simulink model "dcmotor_ff"  (R2014b)
settings: Solver=ode45  StartTime=0.0  StopTime=20  FixedStep=1  RelTol=1e-3
PreLoadFcn:
  | param_dcmotor2
values from neighbouring files (symbols this model uses):
  AngleRange = 3500    [param_dcmotor.m]
  Bm = 1e-4    (= 0.0001)    [param_dcmotor.m]
  FN = 620    [param_dcmotor.m]
  J = 0.028 * 1e-4    (= 2.8e-06)    [param_dcmotor.m]
  KD = 8.20 * 1e-5    (= 8.2e-05)    [param_dcmotor.m]
  Ke = 0.0506    [param_dcmotor.m]
  KI = 0.0291    [param_dcmotor.m]
  KP = 0.0136    [param_dcmotor.m]
  Kt = 0.051    [param_dcmotor.m]
  La = 4.4 * 1e-3    (= 0.0044)    [param_dcmotor.m]
  PWMCycle = 10000    [param_dcmotor.m]
  Ra = 10    [param_dcmotor.m]
  TL = 0    [param_dcmotor.m]
  Vol0 = 2.5    [param_dcmotor.m]
  VolMotor = 24    [param_dcmotor.m]
  VolRange = 4.5    [param_dcmotor.m]
undefined symbols (not defined in the file or in its folder): sigbuilder_block
libraries: simulink x2
settings Model: Creator=yyamamot  LastModifiedBy=kotsuka
settings DataIOCC: SignalLoggingSaveFormat=ModelDataLogs  DSMLogging=off
settings OptimizationCC: ExpressionDepthLimit=2147483647  OptimizeModelRefInitCode=on  LifeSpan=1
settings DebuggingCC: UnderspecifiedInitializationDetection=Classic  MergeDetectMultiDrivingBlocksExec=none  ParameterPrecisionLossMsg=none  FcnCallInpInsideContextMsg=UseLocalSettings  StateNameClashWarn=warning
settings HardwareCC: ProdIntDivRoundTo=Zero  ProdEndianess=LittleEndian  ProdHWDeviceType=Generic->32-bit Embedded Processor
settings RTWCC: SystemTargetFile=ert.tlc  GenCodeOnly=on  TemplateMakefile=ert_default_tmf  Description=Real-Time Workshop Embedded Coder  GenerateReport=on  RTWVerbose=off  ProcessScript=ert_make_rtw_hook  IncludeHyperlinkInReport=on  LaunchReport=on  GenerateTraceInfo=on  GenerateTraceReport=on  GenerateTraceReportSl=on  GenerateTraceReportSf=on  GenerateTraceReportEml=on
settings CodeAppCC: IgnoreCustomStorageClasses=off  CustomSymbolStrType=$N$R$M  InternalIdentifier=Classic
settings ERTTargetCC: GenerateSampleERTMain=on  IncludeMdlTerminateFcn=off  SuppressErrorStatus=on  SupportAbsoluteTime=off  SupportNonFinite=off  SupportComplex=off  ERTCustomFileTemplate=example_file_process.tlc

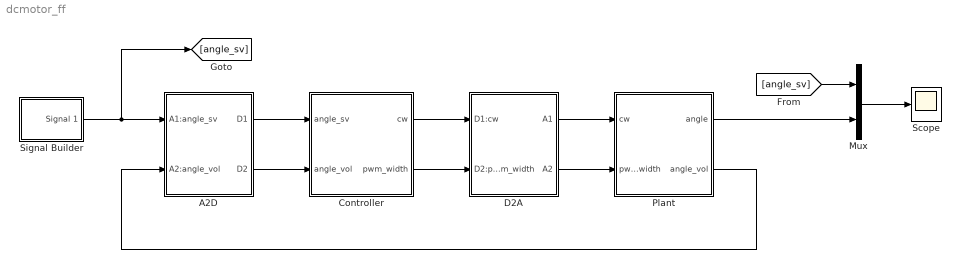
== system dcmotor_ff ==
  A2D : Subsystem
  Controller : Subsystem  TreatAsAtomicUnit=on
  D2A : Subsystem
  Mux : Mux  Inputs=2
  Plant : Subsystem
  Scope : Scope
      settings: YMin=-200  YMax=200
  Signal Builder : Subsystem  Tag=STV Subsys  LoadFcn=sigbuilder_block('load');  StartFcn=sigbuilder_block('start');  StopFcn=sigbuilder_block('stop');  ClipboardFcn=sigbuilder_block('clipboard');  mask(Sigbuilder block){}
      mask help: Simulink:masks:SigbuilderBlock_MD
      mask init:
      | if ~strcmp(get_param(bdroot(gcbh),'SimulationStatus'),'stopped') tuvar = sigbuilder_block('maskInit'); end
      settings: CopyFcn=sigbuilder_block('copy');  DeleteFcn=sigbuilder_block('delete');  ModelCloseFcn=sigbuilder_block('modelClose');  PreSaveFcn=sigbuilder_block('preSave');  PauseFcn=sigbuilder_block('pause');  ContinueFcn=sigbuilder_block('continue');  NameChangeFcn=sigbuilder_block('namechange');  OpenFcn=sigbuilder_block('open',[437.6 199.2 550.4 400 ]);  CloseFcn=sigbuilder_block('close');
      mask Display: plot(0, 0, 100, 100,[2, 2, 32, 32, 2], [68, 8, 8, 68, 68],[32, 2], [38, 38], [32, 19, 2],[53, 60, 44], [32, 17, 17, 2],[16, 16, 31, 31]);txt = getActiveGroup(gcbh);text(2, 100, txt,'verticalAlignment', 'top');
  wires:
  Signal Builder/1(Signal 1) -> A2D/1(A1:angle_sv), [angle_sv]
  Plant/2(angle_vol) -> A2D/2(A2:angle_vol)
  Controller/1(cw) -> D2A/1(D1:cw)
  Controller/2(pwm_width) -> D2A/2(D2:pwm_width)
  D2A/1(A1) -> Plant/1(cw)
  D2A/2(A2) -> Plant/2(pwm_width)
  A2D/1(D1) -> Controller/1(angle_sv)
  A2D/2(D2) -> Controller/2(angle_vol)
  Mux/1 -> Scope/1
  [angle_sv] -> Mux/1
  Plant/1(angle) -> Mux/2

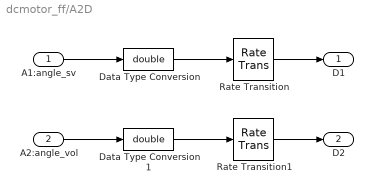
== system dcmotor_ff/A2D ==
  A1:angle_sv : Inport
  A2:angle_vol : Inport  Port=2
  Data Type Conversion : DataTypeConversion  OutDataTypeStr=double
  Data Type Conversion1 : DataTypeConversion  OutDataTypeStr=double
  Rate Transition : RateTransition  Integrity=off  OutPortSampleTime=Ts
  Rate Transition1 : RateTransition  Integrity=off  OutPortSampleTime=Ts
  D1 : Outport
  D2 : Outport  Port=2
  wires:
  A1:angle_sv/1 -> Data Type Conversion/1
  Rate Transition/1 -> D1/1
  Data Type Conversion/1 -> Rate Transition/1
  A2:angle_vol/1 -> Data Type Conversion1/1
  Rate Transition1/1 -> D2/1
  Data Type Conversion1/1 -> Rate Transition1/1

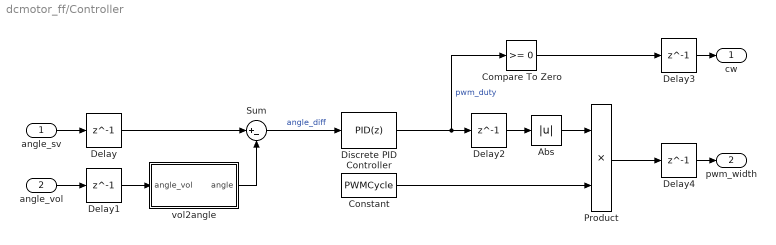
== system dcmotor_ff/Controller ==
  angle_sv : Inport
  angle_vol : Inport  Port=2
  Abs : Abs
  Compare To Zero : simulink/Logic and Bit Operations/Compare To Zero  relop=>=  OutDataTypeStr=uint8
  Constant : Constant  Value=PWMCycle
  Delay{,1..4} (5 alike) : Delay  DelayLength=1
  Discrete PID Controller : simulink/Continuous/PID Controller  Controller=PID  TimeDomain=Discrete-time  SampleTime=-1  IntegratorMethod=Forward Euler  FilterMethod=Forward Euler  Form=Parallel  P=KP  I=KI  D=KD  N=FN  InitialConditionSource=internal  InitialConditionForIntegrator=0  InitialConditionForFilter=0  ExternalReset=none  LimitOutput=on  UpperSaturationLimit=1  LowerSaturationLimit=-1  LinearizeAsGain=off  AntiWindupMode=none  Kb=1  TrackingMode=off  Kt=1  PParamMin=[]  PParamMax=[]  IParamMin=[]  IParamMax=[]  DParamMin=[]  DParamMax=[]  NParamMin=[]  NParamMax=[]  KbParamMin=[]  KbParamMax=[]  KtParamMin=[]  KtParamMax=[]  POutMin=[]  POutMax=[]  IOutMin=[]  IOutMax=[]  DOutMin=[]  DOutMax=[]  NOutMin=[]  NOutMax=[]  KbOutMin=[]  KbOutMax=[]  KtOutMin=[]  KtOutMax=[]  IntegratorOutMin=[]  IntegratorOutMax=[]  FilterOutMin=[]  FilterOutMax=[]  SumOutMin=[]  SumOutMax=[]  SumI1OutMin=[]  SumI1OutMax=[]  SumI2OutMin=[]  SumI2OutMax=[]  SumI3OutMin=[]  SumI3OutMax=[]  SumDOutMin=[]  SumDOutMax=[]  SaturationOutMin=[]  SaturationOutMax=[]  IntegratorContinuousStateAttributes=''  IntegratorStateMustResolveToSignalObject=off  IntegratorRTWStateStorageClass=Auto  FilterContinuousStateAttributes=''  FilterStateMustResolveToSignalObject=off  FilterRTWStateStorageClass=Auto  DifferentiatorICPrevScaledInput=0  DifferentiatorOutMin=[]  DifferentiatorOutMax=[]  UseFilter=on
  Product : Product  RndMeth=Zero
  Sum : Sum  Inputs=|+-
  vol2angle : Subsystem
  cw : Outport
  pwm_width : Outport  Port=2
  wires:
  Product/1 -> Delay4/1
  Discrete PID Controller/1 -> Delay2/1, Compare To Zero/1  "pwm_duty"
  Abs/1 -> Product/1
  Constant/1 -> Product/2
  Sum/1 -> Discrete PID Controller/1  "angle_diff"
  angle_sv/1 -> Delay/1
  angle_vol/1 -> Delay1/1
  vol2angle/1(angle) -> Sum/2
  Compare To Zero/1 -> Delay3/1
  Delay/1 -> Sum/1
  Delay1/1 -> vol2angle/1(angle_vol)
  Delay2/1 -> Abs/1
  Delay3/1 -> cw/1
  Delay4/1 -> pwm_width/1

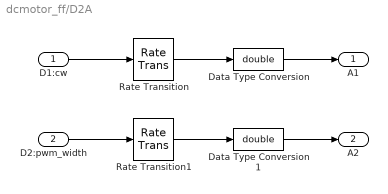
== system dcmotor_ff/D2A ==
  D1:cw : Inport
  D2:pwm_width : Inport  Port=2
  Data Type Conversion : DataTypeConversion  OutDataTypeStr=double
  Data Type Conversion1 : DataTypeConversion  OutDataTypeStr=double
  Rate Transition : RateTransition  Integrity=off  OutPortSampleTime=0
  Rate Transition1 : RateTransition  Integrity=off  OutPortSampleTime=0
  A1 : Outport
  A2 : Outport  Port=2
  wires:
  Rate Transition/1 -> Data Type Conversion/1
  D1:cw/1 -> Rate Transition/1
  Rate Transition1/1 -> Data Type Conversion1/1
  Data Type Conversion1/1 -> A2/1
  D2:pwm_width/1 -> Rate Transition1/1
  Data Type Conversion/1 -> A1/1

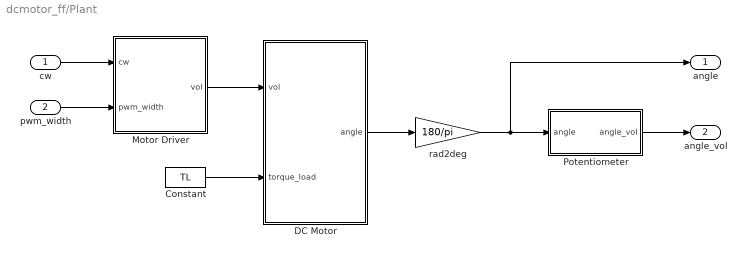
== system dcmotor_ff/Plant ==
  cw : Inport
  pwm_width : Inport  Port=2
  Constant : Constant  Value=TL
  "DC Motor " : Subsystem
  Motor Driver : Subsystem
  Potentiometer : Subsystem
  rad2deg : Gain  Gain=180/pi
  angle : Outport
  angle_vol : Outport  Port=2
  wires:
  Constant/1 -> "DC Motor "/2(torque_load)
  "DC Motor "/1(angle) -> rad2deg/1
  Motor Driver/1(vol) -> "DC Motor "/1(vol)
  pwm_width/1 -> Motor Driver/2(pwm_width)
  Potentiometer/1(angle_vol) -> angle_vol/1
  cw/1 -> Motor Driver/1(cw)
  rad2deg/1 -> Potentiometer/1(angle), angle/1

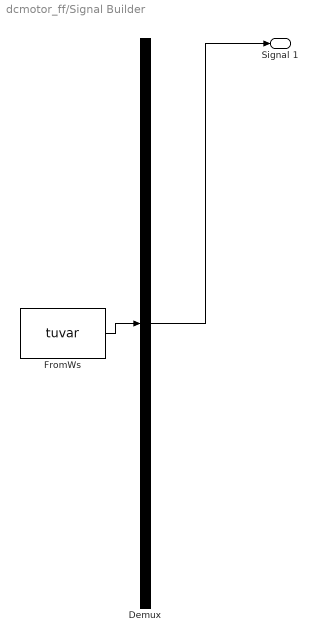
== system dcmotor_ff/Signal Builder ==
  Demux : Demux  Tag=STV Demux  Outputs=1
  FromWs : FromWorkspace  Tag=STV FromWs  VariableName=tuvar  SampleTime=0
      SigBuilderData=|
      | common.afterFinalStr = 'Extrapolate'
      | common.sampleTime = 0
      | dataSet.timeRange = [0 20]
      | dataSet.name = 'Group 1'
      | sbobj.Groups.Name = 'Group 1'
      | sbobj.Groups.Signals.Name = 'Signal 1'
      | sbobj.Groups.Signals.XData = [0 4 4 8 8 12 12 16 16 20]
      | sbobj.Groups.Signals.YData = [0 0 180 180 0 0 -180 -180 0 0]
      | sbobj.Groups.TimeRange = [0 20]
  Signal 1 : Outport  Tag=STV Outport
  wires:
  FromWs/1 -> Demux/1
  Demux/1 -> Signal 1/1

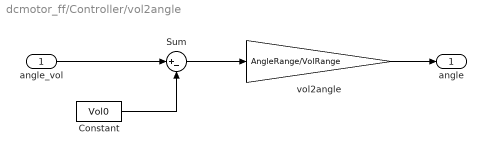
== system dcmotor_ff/Controller/vol2angle ==
  angle_vol : Inport
  Constant : Constant  Value=Vol0
  Sum : Sum  Inputs=|+-
  vol2angle : Gain  Gain=AngleRange/VolRange
  angle : Outport
  wires:
  angle_vol/1 -> Sum/1
  Sum/1 -> vol2angle/1
  vol2angle/1 -> angle/1
  Constant/1 -> Sum/2

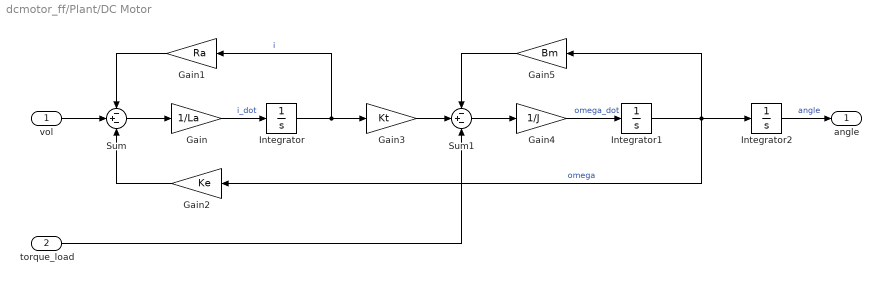
== system dcmotor_ff/Plant/DC Motor  ==
  vol : Inport
  torque_load : Inport  Port=2
  Gain : Gain  Gain=1/La
  Gain1 : Gain  Gain=Ra
  Gain2 : Gain  Gain=Ke
  Gain3 : Gain  Gain=Kt
  Gain4 : Gain  Gain=1/J
  Gain5 : Gain  Gain=Bm
  Integrator : Integrator
  Integrator1 : Integrator
  Integrator2 : Integrator
  Sum : Sum  Inputs=-+-
  Sum1 : Sum  Inputs=-+-
  angle : Outport
  wires:
  Gain/1 -> Integrator/1  "i_dot"
  Integrator/1 -> Gain1/1, Gain3/1  "i"
  Sum/1 -> Gain/1
  Gain1/1 -> Sum/1
  Gain2/1 -> Sum/3
  Gain3/1 -> Sum1/2
  Sum1/1 -> Gain4/1
  Gain4/1 -> Integrator1/1  "omega_dot"
  Integrator1/1 -> Gain5/1, Gain2/1, Integrator2/1  "omega"
  Gain5/1 -> Sum1/1
  torque_load/1 -> Sum1/3
  Integrator2/1 -> angle/1  "angle"
  vol/1 -> Sum/2

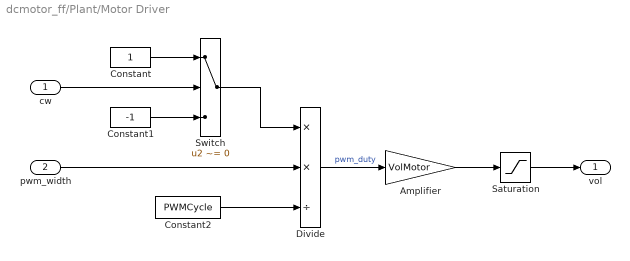
== system dcmotor_ff/Plant/Motor Driver ==
  cw : Inport
  pwm_width : Inport  Port=2
  Amplifier : Gain  Gain=VolMotor
  Constant : Constant
  Constant1 : Constant  Value=-1
  Constant2 : Constant  Value=PWMCycle
  Divide : Product  Inputs=**/
  Saturation : Saturate  UpperLimit=VolMotor  LowerLimit=-VolMotor
  Switch : Switch  Criteria=u2 ~= 0
  vol : Outport
  wires:
  Amplifier/1 -> Saturation/1
  Divide/1 -> Amplifier/1  "pwm_duty"
  cw/1 -> Switch/2
  Constant/1 -> Switch/1
  Constant1/1 -> Switch/3
  Switch/1 -> Divide/1
  pwm_width/1 -> Divide/2
  Constant2/1 -> Divide/3
  Saturation/1 -> vol/1

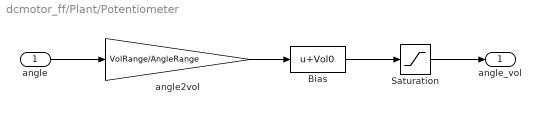
== system dcmotor_ff/Plant/Potentiometer ==
  angle : Inport
  Bias : Bias  Bias=Vol0
  Saturation : Saturate  UpperLimit=Vol0+VolRange/2  LowerLimit=Vol0-VolRange/2
  angle2vol : Gain  Gain=VolRange/AngleRange
  angle_vol : Outport
  wires:
  angle/1 -> angle2vol/1
  angle2vol/1 -> Bias/1
  Bias/1 -> Saturation/1
  Saturation/1 -> angle_vol/1
